simulink model "sys_model"  (R2022b)
settings: Solver=VariableStepAuto  StartTime=0.0  StopTime=10.0  RelTol=1e-3
settings Model: Creator=admin  LastModifiedBy=admin
settings OptimizationCC: ReuseModelBlockBuffer=on
settings RTWCC: GPUComputeCapability=5.0

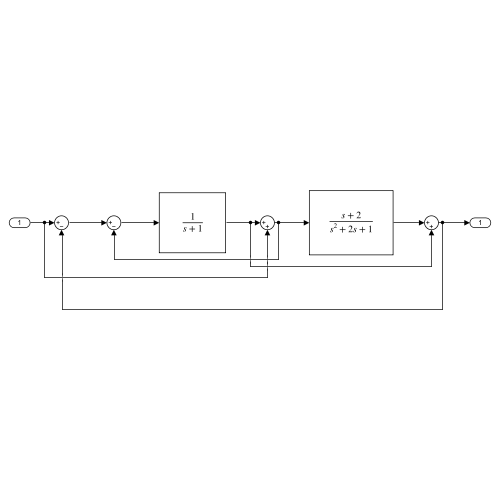
[thumbnail: Simulink's stored preview of the top-level diagram]
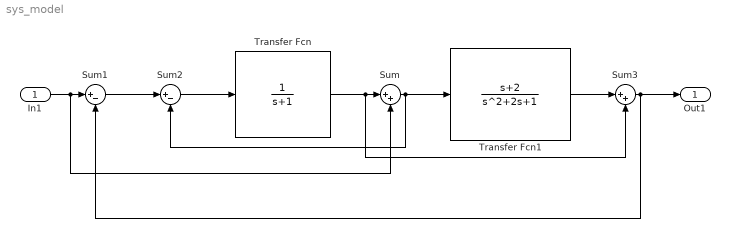
== system sys_model ==
  In1 : Inport
  Sum : Sum  Inputs=|++
  Sum1 : Sum  Inputs=|+-
  Sum2 : Sum  Inputs=|+-
  Sum3 : Sum  Inputs=|++
  Transfer Fcn : TransferFcn  Denominator=[1 1]
  Transfer Fcn1 : TransferFcn  Numerator=[1,2]  Denominator=[1,2,1]
  Out1 : Outport
  wires:
  In1/1 -> Sum/2, Sum1/1
  Sum1/1 -> Sum2/1
  Sum2/1 -> Transfer Fcn/1
  Transfer Fcn/1 -> Sum3/2, Sum/1
  Sum/1 -> Sum2/2, Transfer Fcn1/1
  Transfer Fcn1/1 -> Sum3/1
  Sum3/1 -> Sum1/2, Out1/1
